simulink model "sm_stewart_platform_Identifier_2021Version_desktop"  (R2021b)
settings: Solver=ode4  StartTime=0.0  StopTime=5  FixedStep=0.00001  MaxStep=0.2  RelTol=1e-3  EnableMultiTasking=on
model workspace (MAT data in the model file):
  g_density = 5
values from neighbouring files (symbols this model uses):
  A = -eye(statesSize)*A_scalar    [AL_DNN_main_paper.m]
  c1 = rand(r1, statesSize, statesSize)*0.01    [AL_DNN_main_paper.m]
  c2 = rand(r2, statesSize, 1)*0.1    [AL_DNN_main_paper.m]
  c3 = rand(r3, statesSize, inputSize)*0.1    [AL_DNN_main_paper.m]
  d1 = (rand(r1, statesSize)-0.0)*1    [AL_DNN_main_paper.m]
  d2 = (rand(r2, 1)-0.0)*1    [AL_DNN_main_paper.m]
  d3 = (rand(r3, inputSize)-0.0)*1    [AL_DNN_main_paper.m]
  K1 = eye(statesSize)*1    [AL_DNN_main_paper.m]
  K2 = eye(statesSize)*1    [AL_DNN_main_paper.m]
  K3 = eye(statesSize)*1    [AL_DNN_main_paper.m]
  P_DNN = eye(statesSize)*P_scalar    [AL_DNN_main_paper.m]
  s = zeros(output,ext)    [activation_function.m]
  S = randi(max_noise,[36,1])    [AL_DNN_main_paper.m]
  W10 = (rand(statesSize,r1)-0.5)*0.001    [AL_DNN_main_paper.m]
  W20 = (rand(statesSize,r2)-0.5)*2    [AL_DNN_main_paper.m]
  W30 = (rand(statesSize,r3)-0.5)*2    [AL_DNN_main_paper.m]
  X = systemStates.Data    [AL_DNN_main_paper.m]
  xh0 = (rand(statesSize,1)-0.5)*2    [AL_DNN_main_paper.m]
undefined symbols (not defined in the file or in its folder): B, nom_length, P, Y, Z
libraries: sm_lib x20, sm_stewart_platform_lib x8, nesl_utility x4
(part 3 of 3)

== system sm_stewart_platform_Identifier_2021Version_desktop/Stewart Platform System/Inverse Kinematics Module/Norm 3 ==
  v : Inport
  Dot Product : DotProduct  OutDataTypeStr=Inherit: Inherit via internal rule
  Sqrt : Sqrt  SaturateOnIntegerOverflow=on
  ||v|| : Outport  VectorParamsAs1DForOutWhenUnconnected=off
  wires:
  Dot Product/1 -> Sqrt/1
  Sqrt/1 -> ||v||/1
  v/1 -> Dot Product/1, Dot Product/2

== system sm_stewart_platform_Identifier_2021Version_desktop/Stewart Platform System/Inverse Kinematics Module/Norm 4 ==
  v : Inport
  Dot Product : DotProduct  OutDataTypeStr=Inherit: Inherit via internal rule
  Sqrt : Sqrt  SaturateOnIntegerOverflow=on
  ||v|| : Outport  VectorParamsAs1DForOutWhenUnconnected=off
  wires:
  Dot Product/1 -> Sqrt/1
  Sqrt/1 -> ||v||/1
  v/1 -> Dot Product/1, Dot Product/2

== system sm_stewart_platform_Identifier_2021Version_desktop/Stewart Platform System/Inverse Kinematics Module/Norm 5 ==
  v : Inport
  Dot Product : DotProduct  OutDataTypeStr=Inherit: Inherit via internal rule
  Sqrt : Sqrt  SaturateOnIntegerOverflow=on
  ||v|| : Outport  VectorParamsAs1DForOutWhenUnconnected=off
  wires:
  Dot Product/1 -> Sqrt/1
  Sqrt/1 -> ||v||/1
  v/1 -> Dot Product/1, Dot Product/2

== system sm_stewart_platform_Identifier_2021Version_desktop/Stewart Platform System/Inverse Kinematics Module/Norm 6 ==
  v : Inport
  Dot Product : DotProduct  OutDataTypeStr=Inherit: Inherit via internal rule
  Sqrt : Sqrt  SaturateOnIntegerOverflow=on
  ||v|| : Outport  VectorParamsAs1DForOutWhenUnconnected=off
  wires:
  Dot Product/1 -> Sqrt/1
  Sqrt/1 -> ||v||/1
  v/1 -> Dot Product/1, Dot Product/2

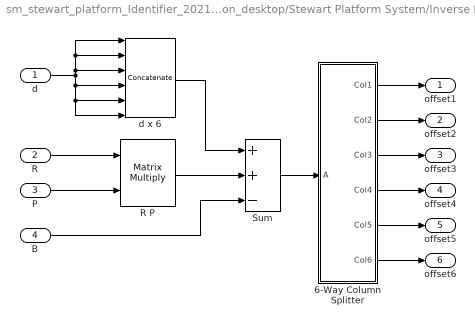
== system sm_stewart_platform_Identifier_2021Version_desktop/Stewart Platform System/Inverse Kinematics Module/Pos Computation ==
  d : Inport
  R : Inport  Port=2
  P : Inport  Port=3
  B : Inport  Port=4
  6-Way Column Splitter : Subsystem
  R P : Product  Multiplication=Matrix(*)  RndMeth=Zero
  Sum : Sum  Inputs=++-
  d x 6 : Concatenate  NumInputs=6  Mode=Multidimensional array  ConcatenateDimension=2
  offset1 : Outport  VectorParamsAs1DForOutWhenUnconnected=off
  offset2 : Outport  Port=2  VectorParamsAs1DForOutWhenUnconnected=off
  offset3 : Outport  Port=3  VectorParamsAs1DForOutWhenUnconnected=off
  offset4 : Outport  Port=4  VectorParamsAs1DForOutWhenUnconnected=off
  offset5 : Outport  Port=5  VectorParamsAs1DForOutWhenUnconnected=off
  offset6 : Outport  Port=6  VectorParamsAs1DForOutWhenUnconnected=off
  wires:
  d/1 -> d x 6/3, d x 6/2, d x 6/1, d x 6/4, d x 6/5, d x 6/6
  Sum/1 -> 6-Way Column Splitter/1(A)
  P/1 -> R P/2
  6-Way Column Splitter/1(Col1) -> offset1/1
  R/1 -> R P/1
  6-Way Column Splitter/2(Col2) -> offset2/1
  6-Way Column Splitter/3(Col3) -> offset3/1
  6-Way Column Splitter/4(Col4) -> offset4/1
  6-Way Column Splitter/5(Col5) -> offset5/1
  6-Way Column Splitter/6(Col6) -> offset6/1
  d x 6/1 -> Sum/1
  B/1 -> Sum/3
  R P/1 -> Sum/2

== system sm_stewart_platform_Identifier_2021Version_desktop/Stewart Platform System/Inverse Kinematics Module/Vel Computation ==
  d' : Inport
  R' : Inport  Port=2
  P : Inport  Port=3
  6-Way Column Splitter : Subsystem
  R P : Product  Multiplication=Matrix(*)  RndMeth=Zero
  Sum : Sum
  d' x 6 : Concatenate  NumInputs=6  Mode=Multidimensional array  ConcatenateDimension=2
  offset1' : Outport  VectorParamsAs1DForOutWhenUnconnected=off
  offset2' : Outport  Port=2  VectorParamsAs1DForOutWhenUnconnected=off
  offset3' : Outport  Port=3  VectorParamsAs1DForOutWhenUnconnected=off
  offset4' : Outport  Port=4  VectorParamsAs1DForOutWhenUnconnected=off
  offset5' : Outport  Port=5  VectorParamsAs1DForOutWhenUnconnected=off
  offset6' : Outport  Port=6  VectorParamsAs1DForOutWhenUnconnected=off
  wires:
  d'/1 -> d' x 6/3, d' x 6/2, d' x 6/1, d' x 6/4, d' x 6/5, d' x 6/6
  Sum/1 -> 6-Way Column Splitter/1(A)
  P/1 -> R P/2
  6-Way Column Splitter/1(Col1) -> offset1'/1
  R'/1 -> R P/1
  6-Way Column Splitter/2(Col2) -> offset2'/1
  6-Way Column Splitter/3(Col3) -> offset3'/1
  6-Way Column Splitter/4(Col4) -> offset4'/1
  6-Way Column Splitter/5(Col5) -> offset5'/1
  6-Way Column Splitter/6(Col6) -> offset6'/1
  d' x 6/1 -> Sum/1
  R P/1 -> Sum/2

== system sm_stewart_platform_Identifier_2021Version_desktop/Stewart Platform System/Manipulator/End Effector ==
  Gripper : Subsystem  mask(Gripper){claw_length=claw_length, claw_width=claw_width, claw_thick=claw_thick, base_thick=base_thick}
      mask prompts: claw_length "Claw Length (cm)"; claw_width "Claw Width (cm)"; claw_thick "Claw Thickness (cm)"; base_thick "Base Thickness (cm)"
      mask help: Models a three-claw robotic gripper. The gripper is completely rigid and for example purposes only.
      mask init:
      | % Compute cross section vertices of gripper base
      | p3 = [+claw_thick / 2; 2 * claw_width];
      | p4 = [-claw_thick / 2; 2 * claw_width];
      | co = cos(2 * pi / 3);
      | si = sin(2 * pi / 3);
      | R = [co +si; -si co];
      | p1 = R * p3;
      | p2 = R * p4;
      | R = [co -si; +si co];
      | p5 = R * p3;
      | p6 = R * p4;
      mask Help:
      | A <em>Gripper</em> models a three-claw robotic gripper.  The gripper is
      | completely rigid and for demonstration purposes only.
      | 
      | The gripper comprises three claws attached to an approximately triangular base.
      | The gripper exposes two frames: the <em>reference</em> frame at the center of the top
      | surface of the base, and the <em>jaw</em> frame at the center of the distil ends
      | of the claws.
      | 
      | <h3>Parameters</h3>
      | 
      | <ul>
      | 
      | <li> <b>Claw Length</b> The length (height) of the trapezoidal claws of the
      |   gripper.  This is the distance between the gripper frame and the top surface of
      |   the gripper base.
      | 
      | <li> <b>Claw Width</b> The width of the trapezoidal claws of the gripper where
      |   they attach to the gripper base.  The claws are narrower at their distal ends.
      |   This value is the main factor determining the size of the gripper base.
      | 
      | <li> <b>Claw Thickness</b> The thickness of the trapezoidal claws of the gripper.
      | 
      | <li> <b>Base Thickness</b> The thickness of the triangular gripper base.
      | 
      | </ul>
      | 
      | <h3>Ports</h3>
      | 
      | <ul>
      | 
      | <li> <b>ref</b> The reference frame of the gripper.  This frame may be used to
      |   connect the gripper to a robot arm.  Its origin is at the center of the top
      |   face of the triangular base, and its z-axis is aligned with the axis of
      |   symmetry of the gripper, pointing up toward the distil ends of the claws.
      | 
      | <li> <b>jaw</b> The jaw frame of the gripper.  The origin of this frame is
      |   centered between the distil ends of the three gripper claws.  The z-axis
      |   points up, aligned with the gripper's axis of symmetry.  The y-axis lies in
      |   the plane of one of the gripper claws.  This frame is often the frame that
      |   a user of a Stewart platform wants to control.
      | 
      | </ul>
      mask Display:
      | image('sm_stewart_platform_gripper.png')
      | color('white')
      | port_label('LConn', 1, 'ref')
      | port_label('RConn', 1, 'jaw')
  Gripper Transform : sm_lib/Frames and Transforms/Rigid Transform  TranslationMethod=StandardAxis  TranslationStandardOffset=grip_height - claw_length  TranslationLengthUnit=cm  TranslationStandardAxis=+Z  TranslationCartesianOffset=[0 0 0]  TranslationROffset=0  TranslationROffsetUnits=m  TranslationZOffset=0  TranslationZOffsetUnits=m  TranslationThetaOffset=0  TranslationThetaOffsetUnits=deg  RotationMethod=None  RotationAngleUnits=deg  RotationStandardAxis=+Z  RotationAngle=0  RotationArbitraryAxis=[0 0 1]  FollAlignAxisA=+X  BaseAlignAxisA=+Y  FollAlignAxisB=+Y  BaseAlignAxisB=+Z  RotationSequenceAxes=FollowerAxes  RotationSequence=XYX  RotationSequenceAngles=[0 0 0]  RotationSequenceAnglesUnits=deg  RotationMatrix=[1 0 0; 0 1 0; 0 0 1]
  Reference Frame : sm_lib/Frames and Transforms/Reference Frame
  Support Shaft : sm_lib/Body Elements/Cylindrical Solid  GraphicAmbientColor=[.1 .1 .1]  BasedOnType=Density  CenterOfMass=[0 0 0]  CenterOfMassUnits=m  GraphicDiffuseColor=[.5 .5 .6]  CylinderLength=grip_height - (claw_length + claw_thick)  CylinderLengthUnits=cm  CylinderRadius=claw_width / 2  CylinderRadiusUnits=cm  Density=g_density  DensityUnits=g/cm^3  DoExposeReferenceFrame=on  GraphicEmissiveColor=[0.0 0.0 0.0]  ExportEntireGeometry=off  SerializedFrames=<Frames/>  MarkerShape=Sphere  MarkerSize=1  GraphicType=FromGeometry  InertiaType=CalculateFromGeometry  Mass=1  MassUnits=kg  MomentsOfInertia=[1 1 1]  MomentsOfInertiaUnits=kg*m^2  GraphicOpacity=1  ProductsOfInertia=[0 0 0]  ProductsOfInertiaUnits=kg*m^2  GraphicShininess=100  GraphicSpecularColor=[.8 .8 1]  GraphicVisPropType=AdvancedVisualProperties
  Support Transform : sm_lib/Frames and Transforms/Rigid Transform  TranslationMethod=StandardAxis  TranslationStandardOffset=(grip_height - (claw_length + claw_thick)) / 2  TranslationLengthUnit=cm  TranslationStandardAxis=+Z  TranslationCartesianOffset=[0 0 0]  TranslationROffset=0  TranslationROffsetUnits=m  TranslationZOffset=0  TranslationZOffsetUnits=m  TranslationThetaOffset=0  TranslationThetaOffsetUnits=deg  RotationMethod=None  RotationAngleUnits=deg  RotationStandardAxis=+Z  RotationAngle=0  RotationArbitraryAxis=[0 0 1]  FollAlignAxisA=+X  BaseAlignAxisA=+Y  FollAlignAxisB=+Y  BaseAlignAxisB=+Z  RotationSequenceAxes=FollowerAxes  RotationSequence=XYX  RotationSequenceAngles=[0 0 0]  RotationSequenceAnglesUnits=deg  RotationMatrix=[1 0 0; 0 1 0; 0 0 1]
  conn : PMIOPort  Side=Right
  grip : PMIOPort  Port=2  Side=Left
  connections:
  Gripper Transform/LConn1 -- Support Transform/LConn1 -- Reference Frame/RConn1 -- conn/RConn1
  Support Shaft/RConn1 -- Support Transform/RConn1
  Gripper/LConn1 -- Gripper Transform/RConn1
  Gripper/RConn1 -- grip/RConn1

== system sm_stewart_platform_Identifier_2021Version_desktop/Stewart Platform System/Noise Generation/Noise S1 ==
  In1 : Inport
  Gain : Gain  Gain=S(1)
  Gain1 : Gain  Gain=S(2)
  Gain2 : Gain  Gain=S(3)
  Product : Product  Inputs=3
  Sin : Trigonometry
  Sin1 : Trigonometry
  Sin2 : Trigonometry
  Out1 : Outport
  wires:
  Product/1 -> Out1/1
  Sin1/1 -> Product/3
  In1/1 -> Gain2/1, Gain1/1, Gain/1
  Sin/1 -> Product/1
  Sin2/1 -> Product/2
  Gain2/1 -> Sin1/1
  Gain/1 -> Sin/1
  Gain1/1 -> Sin2/1

== system sm_stewart_platform_Identifier_2021Version_desktop/Stewart Platform System/Noise Generation/Noise S10 ==
  In1 : Inport
  Gain : Gain  Gain=S(28)
  Gain1 : Gain  Gain=S(29)
  Gain2 : Gain  Gain=S(30)
  Product : Product  Inputs=3
  Sin : Trigonometry
  Sin1 : Trigonometry
  Sin2 : Trigonometry
  Out1 : Outport
  wires:
  Product/1 -> Out1/1
  Sin1/1 -> Product/3
  In1/1 -> Gain2/1, Gain1/1, Gain/1
  Sin/1 -> Product/1
  Sin2/1 -> Product/2
  Gain2/1 -> Sin1/1
  Gain/1 -> Sin/1
  Gain1/1 -> Sin2/1

== system sm_stewart_platform_Identifier_2021Version_desktop/Stewart Platform System/Noise Generation/Noise S11 ==
  In1 : Inport
  Gain : Gain  Gain=S(31)
  Gain1 : Gain  Gain=S(32)
  Gain2 : Gain  Gain=S(33)
  Product : Product  Inputs=3
  Sin : Trigonometry
  Sin1 : Trigonometry
  Sin2 : Trigonometry
  Out1 : Outport
  wires:
  Product/1 -> Out1/1
  Sin1/1 -> Product/3
  In1/1 -> Gain2/1, Gain1/1, Gain/1
  Sin/1 -> Product/1
  Sin2/1 -> Product/2
  Gain2/1 -> Sin1/1
  Gain/1 -> Sin/1
  Gain1/1 -> Sin2/1

== system sm_stewart_platform_Identifier_2021Version_desktop/Stewart Platform System/Noise Generation/Noise S12 ==
  In1 : Inport
  Gain : Gain  Gain=S(34)
  Gain1 : Gain  Gain=S(35)
  Gain2 : Gain  Gain=S(36)
  Product : Product  Inputs=3
  Sin : Trigonometry
  Sin1 : Trigonometry
  Sin2 : Trigonometry
  Out1 : Outport
  wires:
  Product/1 -> Out1/1
  Sin1/1 -> Product/3
  In1/1 -> Gain2/1, Gain1/1, Gain/1
  Sin/1 -> Product/1
  Sin2/1 -> Product/2
  Gain2/1 -> Sin1/1
  Gain/1 -> Sin/1
  Gain1/1 -> Sin2/1

== system sm_stewart_platform_Identifier_2021Version_desktop/Stewart Platform System/Noise Generation/Noise S2 ==
  In1 : Inport
  Gain : Gain  Gain=S(4)
  Gain1 : Gain  Gain=S(5)
  Gain2 : Gain  Gain=S(6)
  Product : Product  Inputs=3
  Sin : Trigonometry
  Sin1 : Trigonometry
  Sin2 : Trigonometry
  Out1 : Outport
  wires:
  Gain1/1 -> Sin2/1
  Gain/1 -> Sin/1
  Gain2/1 -> Sin1/1
  Sin2/1 -> Product/2
  Sin/1 -> Product/1
  In1/1 -> Gain/1, Gain1/1, Gain2/1
  Sin1/1 -> Product/3
  Product/1 -> Out1/1

== system sm_stewart_platform_Identifier_2021Version_desktop/Stewart Platform System/Noise Generation/Noise S3 ==
  In1 : Inport
  Gain : Gain  Gain=S(7)
  Gain1 : Gain  Gain=S(8)
  Gain2 : Gain  Gain=S(9)
  Product : Product  Inputs=3
  Sin : Trigonometry
  Sin1 : Trigonometry
  Sin2 : Trigonometry
  Out1 : Outport
  wires:
  Product/1 -> Out1/1
  Sin1/1 -> Product/3
  In1/1 -> Gain2/1, Gain1/1, Gain/1
  Sin/1 -> Product/1
  Sin2/1 -> Product/2
  Gain2/1 -> Sin1/1
  Gain/1 -> Sin/1
  Gain1/1 -> Sin2/1

== system sm_stewart_platform_Identifier_2021Version_desktop/Stewart Platform System/Noise Generation/Noise S4 ==
  In1 : Inport
  Gain : Gain  Gain=S(10)
  Gain1 : Gain  Gain=S(11)
  Gain2 : Gain  Gain=S(12)
  Product : Product  Inputs=3
  Sin : Trigonometry
  Sin1 : Trigonometry
  Sin2 : Trigonometry
  Out1 : Outport
  wires:
  Product/1 -> Out1/1
  Sin1/1 -> Product/3
  In1/1 -> Gain2/1, Gain1/1, Gain/1
  Sin/1 -> Product/1
  Sin2/1 -> Product/2
  Gain2/1 -> Sin1/1
  Gain/1 -> Sin/1
  Gain1/1 -> Sin2/1

== system sm_stewart_platform_Identifier_2021Version_desktop/Stewart Platform System/Noise Generation/Noise S5 ==
  In1 : Inport
  Gain : Gain  Gain=S(13)
  Gain1 : Gain  Gain=S(14)
  Gain2 : Gain  Gain=S(15)
  Product : Product  Inputs=3
  Sin : Trigonometry
  Sin1 : Trigonometry
  Sin2 : Trigonometry
  Out1 : Outport
  wires:
  Product/1 -> Out1/1
  Sin1/1 -> Product/3
  In1/1 -> Gain2/1, Gain1/1, Gain/1
  Sin/1 -> Product/1
  Sin2/1 -> Product/2
  Gain2/1 -> Sin1/1
  Gain/1 -> Sin/1
  Gain1/1 -> Sin2/1

== system sm_stewart_platform_Identifier_2021Version_desktop/Stewart Platform System/Noise Generation/Noise S6 ==
  In1 : Inport
  Gain : Gain  Gain=S(16)
  Gain1 : Gain  Gain=S(17)
  Gain2 : Gain  Gain=S(18)
  Product : Product  Inputs=3
  Sin : Trigonometry
  Sin1 : Trigonometry
  Sin2 : Trigonometry
  Out1 : Outport
  wires:
  Product/1 -> Out1/1
  Sin1/1 -> Product/3
  In1/1 -> Gain2/1, Gain1/1, Gain/1
  Sin/1 -> Product/1
  Sin2/1 -> Product/2
  Gain2/1 -> Sin1/1
  Gain/1 -> Sin/1
  Gain1/1 -> Sin2/1

== system sm_stewart_platform_Identifier_2021Version_desktop/Stewart Platform System/Noise Generation/Noise S7 ==
  In1 : Inport
  Gain : Gain  Gain=S(19)
  Gain1 : Gain  Gain=S(20)
  Gain2 : Gain  Gain=S(21)
  Product : Product  Inputs=3
  Sin : Trigonometry
  Sin1 : Trigonometry
  Sin2 : Trigonometry
  Out1 : Outport
  wires:
  Product/1 -> Out1/1
  Sin1/1 -> Product/3
  In1/1 -> Gain2/1, Gain1/1, Gain/1
  Sin/1 -> Product/1
  Sin2/1 -> Product/2
  Gain2/1 -> Sin1/1
  Gain/1 -> Sin/1
  Gain1/1 -> Sin2/1

== system sm_stewart_platform_Identifier_2021Version_desktop/Stewart Platform System/Noise Generation/Noise S8 ==
  In1 : Inport
  Gain : Gain  Gain=S(22)
  Gain1 : Gain  Gain=S(23)
  Gain2 : Gain  Gain=S(24)
  Product : Product  Inputs=3
  Sin : Trigonometry
  Sin1 : Trigonometry
  Sin2 : Trigonometry
  Out1 : Outport
  wires:
  Product/1 -> Out1/1
  Sin1/1 -> Product/3
  In1/1 -> Gain2/1, Gain1/1, Gain/1
  Sin/1 -> Product/1
  Sin2/1 -> Product/2
  Gain2/1 -> Sin1/1
  Gain/1 -> Sin/1
  Gain1/1 -> Sin2/1

== system sm_stewart_platform_Identifier_2021Version_desktop/Stewart Platform System/Noise Generation/Noise S9 ==
  In1 : Inport
  Gain : Gain  Gain=S(25)
  Gain1 : Gain  Gain=S(26)
  Gain2 : Gain  Gain=S(27)
  Product : Product  Inputs=3
  Sin : Trigonometry
  Sin1 : Trigonometry
  Sin2 : Trigonometry
  Out1 : Outport
  wires:
  Product/1 -> Out1/1
  Sin1/1 -> Product/3
  In1/1 -> Gain2/1, Gain1/1, Gain/1
  Sin/1 -> Product/1
  Sin2/1 -> Product/2
  Gain2/1 -> Sin1/1
  Gain/1 -> Sin/1
  Gain1/1 -> Sin2/1

== system sm_stewart_platform_Identifier_2021Version_desktop/Stewart Platform System/Inverse Kinematics Module/Pos Computation/6-Way Column Splitter ==
  A : Inport
  Column 1 : Selector  NumberOfDimensions=2  InputPortWidth=3  IndexOptions=Select all,Index vector (dialog)  Indices=-1,1  OutputSizes=1
  Column 2 : Selector  NumberOfDimensions=2  InputPortWidth=3  IndexOptions=Select all,Index vector (dialog)  Indices=-1,2  OutputSizes=1
  Column 3 : Selector  NumberOfDimensions=2  InputPortWidth=3  IndexOptions=Select all,Index vector (dialog)  Indices=-1,3  OutputSizes=1
  Column 4 : Selector  NumberOfDimensions=2  InputPortWidth=3  IndexOptions=Select all,Index vector (dialog)  Indices=-1,4  OutputSizes=1
  Column 5 : Selector  NumberOfDimensions=2  InputPortWidth=3  IndexOptions=Select all,Index vector (dialog)  Indices=-1,5  OutputSizes=1
  Column 6 : Selector  NumberOfDimensions=2  InputPortWidth=3  IndexOptions=Select all,Index vector (dialog)  Indices=-1,6  OutputSizes=1
  Col1 : Outport  VectorParamsAs1DForOutWhenUnconnected=off
  Col2 : Outport  Port=2  VectorParamsAs1DForOutWhenUnconnected=off
  Col3 : Outport  Port=3  VectorParamsAs1DForOutWhenUnconnected=off
  Col4 : Outport  Port=4  VectorParamsAs1DForOutWhenUnconnected=off
  Col5 : Outport  Port=5  VectorParamsAs1DForOutWhenUnconnected=off
  Col6 : Outport  Port=6  VectorParamsAs1DForOutWhenUnconnected=off
  wires:
  A/1 -> Column 3/1, Column 2/1, Column 1/1, Column 4/1, Column 5/1, Column 6/1
  Column 1/1 -> Col1/1
  Column 2/1 -> Col2/1
  Column 3/1 -> Col3/1
  Column 4/1 -> Col4/1
  Column 5/1 -> Col5/1
  Column 6/1 -> Col6/1

== system sm_stewart_platform_Identifier_2021Version_desktop/Stewart Platform System/Inverse Kinematics Module/Vel Computation/6-Way Column Splitter ==
  A : Inport
  Column 1 : Selector  NumberOfDimensions=2  InputPortWidth=3  IndexOptions=Select all,Index vector (dialog)  Indices=-1,1  OutputSizes=1
  Column 2 : Selector  NumberOfDimensions=2  InputPortWidth=3  IndexOptions=Select all,Index vector (dialog)  Indices=-1,2  OutputSizes=1
  Column 3 : Selector  NumberOfDimensions=2  InputPortWidth=3  IndexOptions=Select all,Index vector (dialog)  Indices=-1,3  OutputSizes=1
  Column 4 : Selector  NumberOfDimensions=2  InputPortWidth=3  IndexOptions=Select all,Index vector (dialog)  Indices=-1,4  OutputSizes=1
  Column 5 : Selector  NumberOfDimensions=2  InputPortWidth=3  IndexOptions=Select all,Index vector (dialog)  Indices=-1,5  OutputSizes=1
  Column 6 : Selector  NumberOfDimensions=2  InputPortWidth=3  IndexOptions=Select all,Index vector (dialog)  Indices=-1,6  OutputSizes=1
  Col1 : Outport  VectorParamsAs1DForOutWhenUnconnected=off
  Col2 : Outport  Port=2  VectorParamsAs1DForOutWhenUnconnected=off
  Col3 : Outport  Port=3  VectorParamsAs1DForOutWhenUnconnected=off
  Col4 : Outport  Port=4  VectorParamsAs1DForOutWhenUnconnected=off
  Col5 : Outport  Port=5  VectorParamsAs1DForOutWhenUnconnected=off
  Col6 : Outport  Port=6  VectorParamsAs1DForOutWhenUnconnected=off
  wires:
  A/1 -> Column 3/1, Column 2/1, Column 1/1, Column 4/1, Column 5/1, Column 6/1
  Column 1/1 -> Col1/1
  Column 2/1 -> Col2/1
  Column 3/1 -> Col3/1
  Column 4/1 -> Col4/1
  Column 5/1 -> Col5/1
  Column 6/1 -> Col6/1

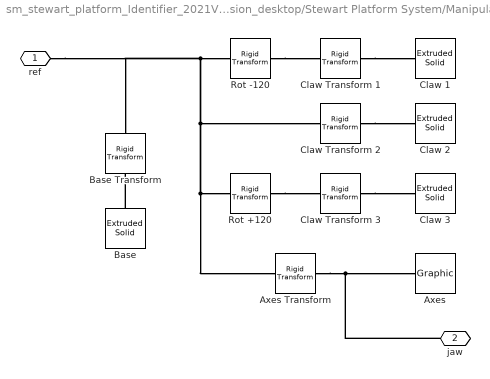
== system sm_stewart_platform_Identifier_2021Version_desktop/Stewart Platform System/Manipulator/End Effector/Gripper ==
  Axes : sm_lib/Body Elements/Graphic  GraphicType=Marker  MarkerShape=Frame  MarkerSize=25  MarkerSizeUnits=m  GraphicVisPropType=SimpleVisualProperties  GraphicDiffuseColor=[0.0 0.0 0.0]  GraphicSpecularColor=[0.2 0.2 0.2]  GraphicAmbientColor=[0.5 0.5 0.5]  GraphicEmissiveColor=[0.0 0.0 0.0 1.0]  GraphicShininess=24.0  GraphicOpacity=1.0
  Axes Transform : sm_lib/Frames and Transforms/Rigid Transform  TranslationMethod=StandardAxis  TranslationStandardOffset=claw_length  TranslationLengthUnit=cm  TranslationStandardAxis=+Z  TranslationCartesianOffset=[0 0 0]  TranslationROffset=0  TranslationROffsetUnits=m  TranslationZOffset=0  TranslationZOffsetUnits=m  TranslationThetaOffset=0  TranslationThetaOffsetUnits=deg  RotationMethod=None  RotationAngleUnits=deg  RotationStandardAxis=+Z  RotationAngle=0  RotationArbitraryAxis=[0 0 1]  FollAlignAxisA=+X  BaseAlignAxisA=+Y  FollAlignAxisB=+Y  BaseAlignAxisB=+Z  RotationSequenceAxes=FollowerAxes  RotationSequence=XYX  RotationSequenceAngles=[0 0 0]  RotationSequenceAnglesUnits=deg  RotationMatrix=[1 0 0; 0 1 0; 0 0 1]
  Base : sm_lib/Body Elements/Extruded Solid  GraphicAmbientColor=[0.1 0.1 0]  BasedOnType=Density  CenterOfMass=[0 0 0]  CenterOfMassUnits=m  GraphicDiffuseColor=[0.9 0.75 0] * 0.8  ExportConvexHullGeometry=off  ExtrusionCrossSection=[p1 p2 p3 p4 p5 p6]'  ExtrusionCrossSectionUnits=cm  Density=g_density  DensityUnits=g/cm^3  DoExposeReferenceFrame=on  GraphicEmissiveColor=[0.0 0.0 0.0]  ExportEntireGeometry=off  ExtrusionLength=base_thick  ExtrusionLengthUnits=cm  ExtrusionType=General  SerializedFrames=<Frames/>  MarkerShape=Sphere  MarkerSize=1  GraphicType=FromGeometry  InertiaType=CalculateFromGeometry  Mass=1  MassUnits=kg  MomentsOfInertia=[1 1 1]  MomentsOfInertiaUnits=kg*m^2  PolygonNumSides=1  GraphicOpacity=1  PolygonOuterRadius=1  PolygonOuterRadiusUnits=m  ProductsOfInertia=[0 0 0]  ProductsOfInertiaUnits=kg*m^2  GraphicShininess=80  GraphicSpecularColor=[0.9 0.75 0] * 0.8  GraphicVisPropType=AdvancedVisualProperties
  Base Transform : sm_lib/Frames and Transforms/Rigid Transform  TranslationMethod=StandardAxis  TranslationStandardOffset=base_thick / 2  TranslationLengthUnit=cm  TranslationStandardAxis=-Z  TranslationCartesianOffset=[0 0 0]  TranslationROffset=0  TranslationROffsetUnits=m  TranslationZOffset=0  TranslationZOffsetUnits=m  TranslationThetaOffset=0  TranslationThetaOffsetUnits=deg  RotationMethod=None  RotationAngleUnits=deg  RotationStandardAxis=+Z  RotationAngle=0  RotationArbitraryAxis=[0 0 1]  FollAlignAxisA=+X  BaseAlignAxisA=+Y  FollAlignAxisB=+Y  BaseAlignAxisB=+Z  RotationSequenceAxes=FollowerAxes  RotationSequence=XYX  RotationSequenceAngles=[0 0 0]  RotationSequenceAnglesUnits=deg  RotationMatrix=[1 0 0; 0 1 0; 0 0 1]
  Claw 1 : sm_lib/Body Elements/Extruded Solid  GraphicAmbientColor=[0.3 0.3 0]  BasedOnType=Density  CenterOfMass=[0 0 0]  CenterOfMassUnits=m  GraphicDiffuseColor=[0.9 0.75 0]  ExportConvexHullGeometry=off  ExtrusionCrossSection=[0 0; claw_width 0; claw_width/3 claw_length; 0 claw_length]  ExtrusionCrossSectionUnits=cm  Density=g_density  DensityUnits=g/cm^3  DoExposeReferenceFrame=on  GraphicEmissiveColor=[0.0 0.0 0.0]  ExportEntireGeometry=off  ExtrusionLength=claw_thick  ExtrusionLengthUnits=cm  ExtrusionType=General  SerializedFrames=<Frames/>  MarkerShape=Sphere  MarkerSize=1  GraphicType=FromGeometry  InertiaType=CalculateFromGeometry  Mass=1  MassUnits=kg  MomentsOfInertia=[1 1 1]  MomentsOfInertiaUnits=kg*m^2  PolygonNumSides=1  GraphicOpacity=1  PolygonOuterRadius=1  PolygonOuterRadiusUnits=m  ProductsOfInertia=[0 0 0]  ProductsOfInertiaUnits=kg*m^2  GraphicShininess=120  GraphicSpecularColor=[0.9 0.75 0]  GraphicVisPropType=AdvancedVisualProperties
  Claw 2 : sm_lib/Body Elements/Extruded Solid  GraphicAmbientColor=[0.3 0.3 0]  BasedOnType=Density  CenterOfMass=[0 0 0]  CenterOfMassUnits=m  GraphicDiffuseColor=[0.9 0.75 0]  ExportConvexHullGeometry=off  ExtrusionCrossSection=[0 0; claw_width 0; claw_width/3 claw_length; 0 claw_length]  ExtrusionCrossSectionUnits=cm  Density=g_density  DensityUnits=g/cm^3  DoExposeReferenceFrame=on  GraphicEmissiveColor=[0.0 0.0 0.0]  ExportEntireGeometry=off  ExtrusionLength=claw_thick  ExtrusionLengthUnits=cm  ExtrusionType=General  SerializedFrames=<Frames/>  MarkerShape=Sphere  MarkerSize=1  GraphicType=FromGeometry  InertiaType=CalculateFromGeometry  Mass=1  MassUnits=kg  MomentsOfInertia=[1 1 1]  MomentsOfInertiaUnits=kg*m^2  PolygonNumSides=1  GraphicOpacity=1  PolygonOuterRadius=1  PolygonOuterRadiusUnits=m  ProductsOfInertia=[0 0 0]  ProductsOfInertiaUnits=kg*m^2  GraphicShininess=120  GraphicSpecularColor=[0.9 0.75 0]  GraphicVisPropType=AdvancedVisualProperties
  Claw 3 : sm_lib/Body Elements/Extruded Solid  GraphicAmbientColor=[0.3 0.3 0]  BasedOnType=Density  CenterOfMass=[0 0 0]  CenterOfMassUnits=m  GraphicDiffuseColor=[0.9 0.75 0]  ExportConvexHullGeometry=off  ExtrusionCrossSection=[0 0; claw_width 0; claw_width/3 claw_length; 0 claw_length]  ExtrusionCrossSectionUnits=cm  Density=g_density  DensityUnits=g/cm^3  DoExposeReferenceFrame=on  GraphicEmissiveColor=[0.0 0.0 0.0]  ExportEntireGeometry=off  ExtrusionLength=claw_thick  ExtrusionLengthUnits=cm  ExtrusionType=General  SerializedFrames=<Frames/>  MarkerShape=Sphere  MarkerSize=1  GraphicType=FromGeometry  InertiaType=CalculateFromGeometry  Mass=1  MassUnits=kg  MomentsOfInertia=[1 1 1]  MomentsOfInertiaUnits=kg*m^2  PolygonNumSides=1  GraphicOpacity=1  PolygonOuterRadius=1  PolygonOuterRadiusUnits=m  ProductsOfInertia=[0 0 0]  ProductsOfInertiaUnits=kg*m^2  GraphicShininess=120  GraphicSpecularColor=[0.9 0.75 0]  GraphicVisPropType=AdvancedVisualProperties
  Claw Transform 1 : sm_lib/Frames and Transforms/Rigid Transform  TranslationMethod=StandardAxis  TranslationStandardOffset=claw_width  TranslationLengthUnit=cm  TranslationStandardAxis=+Y  TranslationCartesianOffset=[0 0 0]  TranslationROffset=0  TranslationROffsetUnits=m  TranslationZOffset=0  TranslationZOffsetUnits=m  TranslationThetaOffset=0  TranslationThetaOffsetUnits=deg  RotationMethod=AlignedAxes  RotationAngleUnits=deg  RotationStandardAxis=+Z  RotationAngle=0  RotationArbitraryAxis=[0 0 1]  FollAlignAxisA=+X  BaseAlignAxisA=+Y  FollAlignAxisB=+Y  BaseAlignAxisB=+Z  RotationSequenceAxes=FollowerAxes  RotationSequence=XYX  RotationSequenceAngles=[0 0 0]  RotationSequenceAnglesUnits=deg  RotationMatrix=[1 0 0; 0 1 0; 0 0 1]
  Claw Transform 2 : sm_lib/Frames and Transforms/Rigid Transform  TranslationMethod=StandardAxis  TranslationStandardOffset=claw_width  TranslationLengthUnit=cm  TranslationStandardAxis=+Y  TranslationCartesianOffset=[0 0 0]  TranslationROffset=0  TranslationROffsetUnits=m  TranslationZOffset=0  TranslationZOffsetUnits=m  TranslationThetaOffset=0  TranslationThetaOffsetUnits=deg  RotationMethod=AlignedAxes  RotationAngleUnits=deg  RotationStandardAxis=+Z  RotationAngle=0  RotationArbitraryAxis=[0 0 1]  FollAlignAxisA=+X  BaseAlignAxisA=+Y  FollAlignAxisB=+Y  BaseAlignAxisB=+Z  RotationSequenceAxes=FollowerAxes  RotationSequence=XYX  RotationSequenceAngles=[0 0 0]  RotationSequenceAnglesUnits=deg  RotationMatrix=[1 0 0; 0 1 0; 0 0 1]
  Claw Transform 3 : sm_lib/Frames and Transforms/Rigid Transform  TranslationMethod=StandardAxis  TranslationStandardOffset=claw_width  TranslationLengthUnit=cm  TranslationStandardAxis=+Y  TranslationCartesianOffset=[0 0 0]  TranslationROffset=0  TranslationROffsetUnits=m  TranslationZOffset=0  TranslationZOffsetUnits=m  TranslationThetaOffset=0  TranslationThetaOffsetUnits=deg  RotationMethod=AlignedAxes  RotationAngleUnits=deg  RotationStandardAxis=+Z  RotationAngle=0  RotationArbitraryAxis=[0 0 1]  FollAlignAxisA=+X  BaseAlignAxisA=+Y  FollAlignAxisB=+Y  BaseAlignAxisB=+Z  RotationSequenceAxes=FollowerAxes  RotationSequence=XYX  RotationSequenceAngles=[0 0 0]  RotationSequenceAnglesUnits=deg  RotationMatrix=[1 0 0; 0 1 0; 0 0 1]
  Rot +120 : sm_lib/Frames and Transforms/Rigid Transform  TranslationMethod=None  TranslationStandardOffset=0  TranslationLengthUnit=m  TranslationStandardAxis=+Z  TranslationCartesianOffset=[0 0 0]  TranslationROffset=0  TranslationROffsetUnits=m  TranslationZOffset=0  TranslationZOffsetUnits=m  TranslationThetaOffset=0  TranslationThetaOffsetUnits=deg  RotationMethod=StandardAxis  RotationAngleUnits=deg  RotationStandardAxis=+Z  RotationAngle=+120  RotationArbitraryAxis=[0 0 1]  FollAlignAxisA=+X  BaseAlignAxisA=+Y  FollAlignAxisB=+Y  BaseAlignAxisB=+Z  RotationSequenceAxes=FollowerAxes  RotationSequence=XYX  RotationSequenceAngles=[0 0 0]  RotationSequenceAnglesUnits=deg  RotationMatrix=[1 0 0; 0 1 0; 0 0 1]
  Rot -120 : sm_lib/Frames and Transforms/Rigid Transform  TranslationMethod=None  TranslationStandardOffset=0  TranslationLengthUnit=m  TranslationStandardAxis=+Z  TranslationCartesianOffset=[0 0 0]  TranslationROffset=0  TranslationROffsetUnits=m  TranslationZOffset=0  TranslationZOffsetUnits=m  TranslationThetaOffset=0  TranslationThetaOffsetUnits=deg  RotationMethod=StandardAxis  RotationAngleUnits=deg  RotationStandardAxis=+Z  RotationAngle=-120  RotationArbitraryAxis=[0 0 1]  FollAlignAxisA=+X  BaseAlignAxisA=+Y  FollAlignAxisB=+Y  BaseAlignAxisB=+Z  RotationSequenceAxes=FollowerAxes  RotationSequence=XYX  RotationSequenceAngles=[0 0 0]  RotationSequenceAnglesUnits=deg  RotationMatrix=[1 0 0; 0 1 0; 0 0 1]
  ref : PMIOPort  Side=Left
  jaw : PMIOPort  Port=2  Side=Right
  connections:
  Claw Transform 1/RConn1 -- Claw 1/RConn1
  Claw Transform 2/LConn1 -- ref/RConn1 -- Base Transform/LConn1 -- Rot -120/LConn1 -- Axes Transform/LConn1 -- Rot +120/LConn1
  Claw Transform 2/RConn1 -- Claw 2/RConn1
  Claw Transform 3/RConn1 -- Claw 3/RConn1
  Base/RConn1 -- Base Transform/RConn1
  Axes Transform/RConn1 -- Axes/RConn1 -- jaw/RConn1
  Rot -120/RConn1 -- Claw Transform 1/LConn1
  Rot +120/RConn1 -- Claw Transform 3/LConn1

== matlab function sm_stewart_platform_Identifier_2021Version_desktop/Stewart Platform System/Pseudolineal/MATLAB Function1 ==
  data: x input; y output; c input; d input
function y = fcn(x, c, d)
[output,input,ext] = size(c);
s = zeros(output,ext);
for i = 1:ext
    for j = 1:output
        z = 0;
        for k = 1:input
            z = z + x(k,1)*c(j,k,i);
        end
        s(j,i) = 1/(1+exp(-z));
    end
end

y = s + d;

== matlab function sm_stewart_platform_Identifier_2021Version_desktop/Stewart Platform System/Pseudolineal/MATLAB Function ==
  data: x input; y output; c input; d input
function y = fcn(x, c, d)
[output,input,ext] = size(c);
s = zeros(output,ext);
for i = 1:ext
    for j = 1:output
        z = 0;
        for k = 1:input
            z = z + x(k,1)*c(j,k,i);
        end
        s(j,i) = 1/(1+exp(-z));
    end
end

y = s + d;

== matlab function sm_stewart_platform_Identifier_2021Version_desktop/Stewart Platform System/Pseudolineal/MATLAB Function2 ==
  data: x input; y output; c input; d input
function y = fcn(x, c, d)
[output,input,ext] = size(c);
s = zeros(output,ext);
for i = 1:ext
    for j = 1:output
        z = 0;
        for k = 1:input
            z = z + x(k,1)*c(j,k,i);
        end
        s(j,i) = 1/(1+exp(-z));
    end
end

y = s + d;

== matlab function sm_stewart_platform_Identifier_2021Version_desktop/Stewart Platform System/DNN/MATLAB Function1 ==
  data: x input; y output; c input; d input
function y = fcn(x, c, d)
[output,input,ext] = size(c);
s = zeros(output,ext);
for i = 1:ext
    for j = 1:output
        z = 0;
        for k = 1:input
            z = z + x(k,1)*c(j,k,i);
        end
        s(j,i) = 1/(1+exp(-z));
    end
end

y = s + d;

== matlab function sm_stewart_platform_Identifier_2021Version_desktop/Stewart Platform System/DNN/MATLAB Function2 ==
  data: x input; y output; c input; d input
function y = fcn(x, c, d)
[output,input,ext] = size(c);
s = zeros(output,ext);
for i = 1:ext
    for j = 1:output
        z = 0;
        for k = 1:input
            z = z + x(k,1)*c(j,k,i);
        end
        s(j,i) = 1/(1+exp(-z));
    end
end

y = s + d;

== matlab function sm_stewart_platform_Identifier_2021Version_desktop/Stewart Platform System/Pseudolineal/MATLAB Function3 ==
  data: A input; y output; e output
function [y, e] = fcn(A)
% This funciton evaluates if all eigenvalues of the matrix A are negatvies
% for stability purposes

% Add elements for saving the eigenvalues


% Obtain eigenvalues
e = eig(A);
% Size of A matrix
e_length = length(e);
cont = 0;
for i = 1:e_length
    % Evaluate condition
    if e(i) < 0
        cont = cont + 1;
    end
end

% Verifiy negative eigenvalues number
if cont == e_length
    h = 1;
else
    h = 0;
end
y = h;
